simulink model "UAV_sync_known_sim_wrong_version"  (R2018b)
settings: Solver=ode23tb  StartTime=0.0  StopTime=35
values from neighbouring files (symbols this model uses):
  C_rho = 1.225    [SC42120_UAV_Preconditions.m]
  D0 = [M0 0 0 0 0 0 ... (first row only)    [SC42120_UAV_Preconditions.m]
  D1 = [eye(3)*M1 zeros(3,3) ... (first row only)    [UAV_sync_known.m]    (also in UAV_sync_unknown.m; UAV_sync_unknown_gap.m)
  D2 = [eye(3)*M2 zeros(3,3) ... (first row only)    [UAV_sync_known.m]    (also in UAV_sync_unknown.m; UAV_sync_unknown_gap.m)
  Derivative_gain_phi = 50    [SC42120_UAV_Preconditions.m]
  Derivative_gain_psi = 50    [SC42120_UAV_Preconditions.m]
  Derivative_gain_theta = 50    [SC42120_UAV_Preconditions.m]
  Derivative_gain_x = 50    [SC42120_UAV_Preconditions.m]
  Derivative_gain_y = 50    [SC42120_UAV_Preconditions.m]
  Derivative_gain_z = 50    [SC42120_UAV_Preconditions.m]
  G = 9.80665    [SC42120_UAV_Preconditions.m]
  g0 = [0;0;-M0*G;0;0;0]    [SC42120_UAV_Preconditions.m]
  I0 = [0.02 0 -0.01 ... (first row only)    [SC42120_UAV_Preconditions.m]
  I1 = [0.1 0 -0.01 ... (first row only)    [UAV_sync_known.m]    (also in UAV_sync_unknown.m; UAV_sync_unknown_gap.m)
  I2 = 2*[0.1 0 -0.01 ... (first row only)    [UAV_sync_known.m]    (also in UAV_sync_unknown.m; UAV_sync_unknown_gap.m)
  InitWind = [0;0;0]    [SC42120_UAV_Preconditions.m]
  Kp = diag(P)    [SC42120_UAV_Preconditions.m]
  Kv = diag(V)    [SC42120_UAV_Preconditions.m]
  M0 = 10    [SC42120_UAV_Preconditions.m]
  M1 = 20    [UAV_sync_known.m]    (also in UAV_sync_unknown.m; UAV_sync_unknown_gap.m)
  M2 = 30    [UAV_sync_known.m]    (also in UAV_sync_unknown.m; UAV_sync_unknown_gap.m)
  Proportional_phi = 50    [SC42120_UAV_Preconditions.m]
  Proportional_psi = 50    [SC42120_UAV_Preconditions.m]
  Proportional_theta = 50    [SC42120_UAV_Preconditions.m]
  Proportional_x = 50    [SC42120_UAV_Preconditions.m]
  Proportional_y = 50    [SC42120_UAV_Preconditions.m]
  Proportional_z = 50    [SC42120_UAV_Preconditions.m]
undefined symbols (not defined in the file or in its folder): Aero, APlane, Bxl, C, Ctr, deg, DiscIntNeverNeededParam, F, Guid, Init, Light, MIL, Path, rad, s, Trim, Utility
libraries: aerolibconvert2 x37, simulink x15, dspsigops x7, shared6dof x4, aerolibasang x4, sharedutil x4, simulink_extras x3, aerolibadyn x1, aerolibtransform2 x1, aerolibwind2 x1
(part 6 of 6)

== matlab function UAV_sync_known_sim_wrong_version/Node 0/VF Approach/AUTOPILOT/Low-level Controllers/Pitch controller/TRASH/Pitch_PID_MATLAB_Fcn ==
  data: desired_rate input; meas_pitch_rate input; out output; meas_roll_angle input; scaler input; aspeed input; time input; parteInt output; parteDer output; parteFF output; parteP output; parameters input
function [out, parteInt, parteDer, parteFF, parteP] = pitch_rate_controller...
    (desired_rate, meas_pitch_rate, meas_roll_angle, scaler, aspeed, time, ... % inputs
    parameters) % parameters
%%

gainstau = parameters(1);
gainsP = parameters(2);
gainsI = parameters(3);
gainsD = parameters(4);
gainsimax = parameters(5);
gainsFF = parameters(6);
airspeed_min = parameters(7);
eas2tas = parameters(8);
roll_limit = parameters(9);

persistent last_t;
persistent last_out;
persistent pidInfoI;

if isempty(last_t)
    last_t = 0;
end

if isempty(pidInfoI)
    pidInfoI = 0;
end

if isempty(last_out)
    last_out = 0;
end

if time==0
    last_t = 0;
    last_out=0;
    pidInfoI=0;
end

%% Start of code

tnow = time;
dt = tnow - last_t;

if (last_t == 0 || dt > 1)
    dt = 0;
end

last_t = tnow;

delta_time = dt; % * 0.001; Because the microcontroller gives [ms] - REMOVED

achieved_rate = meas_pitch_rate;
rate_error = rad2deg((desired_rate - achieved_rate) * scaler);

if gainsI > 0
    k_I = gainsI;
        if (gainsFF == 0)
    %                     /*
    %               if the user hasn't set a direct FF then assume they are
    %               not doing sophisticated tuning. Set a minimum I value of
    %               0.15 to ensure that the time constant for trimming in
    %               pitch is not too long. We have had a lot of user issues
    %               with very small I value leading to very slow pitch
    %               trimming, which causes a lot of problems for TECS. A
    %               value of 0.15 is still quite small, but a lot better
    %               than what many users are running.
    %              */
            k_I = max(k_I, 0.15);
        end
    ki_rate = k_I * gainstau;
    %     only integrate if gain and time step are positive and airspeed above min value.
    if (dt > 0 && aspeed > 0.5*airspeed_min)
        integrator_delta = rate_error * ki_rate * delta_time * scaler;
        if last_out < -45
            %              prevent the integrator from increasing if surface defln demand is above the upper limit
            integrator_delta = max(integrator_delta, 0);
        elseif last_out > 45
            %             prevent the integrator from decreasing if surface defln demand  is below the lower limit
            integrator_delta = min(integrator_delta, 0);
        end
        pidInfoI = pidInfoI + integrator_delta;
    end
else
    pidInfoI = 0;
end

intLimScaled = gainsimax * 0.01;
pidInfoI = constrain_value(pidInfoI, -intLimScaled, intLimScaled);


% get ESTIMATED to TRUE airspeed ratio (assuming 1, as in
% Airspeed_calibration.cpp)

% Calculate equivalent gains so that values for K_P and K_I can be taken across from the old PID law
% No conversion is required for K_D
kp_ff = max((gainsP - gainsI * gainstau) * gainstau  - gainsD , 0) / eas2tas;
k_ff = gainsFF / eas2tas;

% Calculate the demanded control surface deflection
% Note the scaler is applied again. We want a 1/speed scaler applied to the feed-forward
% path, but want a 1/speed^2 scaler applied to the rate error path.
% This is because acceleration scales with speed^2, but rate scales with speed.
pidInfoD = rate_error * gainsD * scaler;
pidInfoP = desired_rate * kp_ff * scaler;
pidInfoFF = desired_rate * k_ff * scaler;
last_out = pidInfoFF + pidInfoP + pidInfoD;
% pidInfodesired = desired_rate;
last_out = last_out + pidInfoI;

% when we are past the users defined roll limit for the
% aircraft our priority should be to bring the aircraft back
% within the roll limit. Using elevator for pitch control at
% large roll angles is ineffective, and can be counter
% productive as it induces earth-frame yaw which can reduce
% the ability to roll. We linearly reduce elevator input when
% beyond the configured roll limit, reducing to zero at 90
% degrees
roll_wrapped = rad2deg(abs(meas_roll_angle));

if roll_wrapped > 90
    roll_wrapped = 180-roll_wrapped;
end
% 
% if (roll_wrapped>roll_limit+5 && roll_limit<85 && abs(meas_pitch_rate) < 70)
%     roll_prop = (roll_wrapped - (roll_limit+5) / (90-roll_limit));
%     last_out = last_out * (1 - roll_prop);
% end

out = constrain_value(last_out * 100, -4500, 4500);

parteInt = pidInfoI;
parteDer = pidInfoD;
parteFF = pidInfoFF;
parteP = pidInfoP;

== matlab function UAV_sync_known_sim_wrong_version/Node 0/VF Approach/BIXLER DYNAMICS/RUBBISH BIN/Straight Line/Vg Estimator/SL_Estimator ==
  data: chi input; chi_d input; chi_q input; e input; Vg_hat input; Vg_hat_dot output size=1; param input; e output; f1 output; f2 output; Vg input
function [Vg_hat_dot, e, f1, f2]...
    = estimator (chi, chi_d, chi_q, e, Vg_hat, param, Vg)
%  feedback, der, term2, last_term,diff_chi, diff_2,
%estimator of Vg'
%% Parameters
y_int = param(1);
W = param(2);
Va = param(3);
epsi = param(4);
phiw = param(5);
chi_inf = param(6);
k = param(7);
kk=param(8);
Gamma = param(9);
sigma = param(10);

%% Law

rho = y_int^2/pi^2;   % Positive scale factor used to weight the terms so that y and chi are similar in magnitude

diff_chi = chi-chi_d; % Error of course angle

term =diff_chi/epsi;
if abs(term)<=1
    sat=term;
else
    sat=sign(term);
end

% % derivative of Vg' over x'
der = W*sin(phiw-chi)+(Va^2-W^2*(sin(phiw-chi))^2)^(-0.5)*W^2*sin(phiw-chi)*cos(phiw-chi); % partial derivative of Vg' over chi'
% 
% % Vg2_hat_dot =-i*Gamma*rho*diff_chi*chi_inf*2/pi*(k*(sin(chi2)-a*cos(chi2)))/(1+(k*(e))^2)+der*(i*chi_inf*2/pi*(k*(sin(chi2)-a*cos(chi2)))/(1+(k*(e))^2)*Vg2_hat-kk*sat);
term2 = (-1*chi_inf*2/pi*(k*sin(chi - chi_q))/(1+(k*(e))^2)*Vg_hat);
last_term = -1*kk*sat;
f2 = (sin(chi - chi_q));
f1 =  k/(1+(k*e)^2)*Gamma*rho*diff_chi*chi_inf*2/pi;

alpha = 0.4578;

% if Vg_hat - Vg > 0.5
%     sigma = (Vg_hat - Vg);
% else
%     sigma = 0;
% end
Gamma = 5;
Vg_hat_dot = Gamma/alpha*rho*diff_chi*chi_inf*2/pi*(k*(sin(chi-chi_q)))/(1+(k*(e))^2)...
    - sigma* Gamma * Vg_hat +...
     1*der*(term2/alpha +last_term);



end

== matlab function UAV_sync_known_sim_wrong_version/Node 0/VF Approach/AUTOPILOT/Low-level Controllers/Pitch controller/TRASH/Coordination_offset_MATLAB_Fcn ==
  data: bank_angle input; rate_offset output; meas_pitch_angle input; aspeed input; parameters input; inverted output
function [rate_offset, inverted] = coord_rate_offset(bank_angle, meas_pitch_angle, aspeed, parameters)

param = [  parameters(1), parameters(2), parameters(3), parameters(4) ];
[rate_offset, inverted] = get_coordination_rate(bank_angle, meas_pitch_angle, aspeed, param);

== matlab function UAV_sync_known_sim_wrong_version/Node 0/VF Approach/BIXLER DYNAMICS/RUBBISH BIN/TECS/Energy calculations/Calculate energies/TAS Rate Limiter ==
  data: TS_dem_adj output; TAS_dem input; TAS_rate_dem output; velRateMax input; velRateMin input
function [TS_dem_adj, TAS_rate_dem] = RateLimiter (TAS_dem, velRateMax, velRateMin)

persistent TAS_dem_adj
persistent TAS_dem_last

TASmin = 6;
TASmax = 35;

if isempty(TAS_dem_adj)
    TAS_dem_adj = 0;
end

if isempty(TAS_dem_last)
    TAS_dem_last = 0;
end


% Apply rate limit
if ((TAS_dem - TAS_dem_adj) > (velRateMax * 0.1))
    TAS_dem_adj = TAS_dem_adj + velRateMax * 0.1;
    TAS_rate_dem = velRateMax;
elseif ((TAS_dem - TAS_dem_adj) < (velRateMin * 0.1))
    TAS_dem_adj = TAS_dem_adj + velRateMin * 0.1;
    TAS_rate_dem = velRateMin;
else
    TAS_dem_adj = TAS_dem;
    TAS_rate_dem = (TAS_dem - TAS_dem_last) / 0.1;
end
%     Constrain speed demand again to protect against bad values on initialisation.
TAS_dem_adj = constrain_value(TAS_dem_adj, TASmin, TASmax);

TS_dem_adj = TAS_dem_adj; % Output 
TAS_dem_last = TAS_dem;

== matlab function UAV_sync_known_sim_wrong_version/Node 0/VF Approach/BIXLER DYNAMICS/RUBBISH BIN/TECS/PITCH1/Integrator ==
  data: integSEB_delta input; y output; integSEB_min input; integSEB_max input
function y = fcn(integSEB_delta, integSEB_min, integSEB_max)

persistent integSEB_state

if isempty(integSEB_state)
    integSEB_state = 0;
end

integSEB_state = constrain_value(integSEB_state + integSEB_delta, integSEB_min, integSEB_max);

y = integSEB_state;

== matlab function UAV_sync_known_sim_wrong_version/Node 0/VF Approach/BIXLER DYNAMICS/RUBBISH BIN/Straight Line/Compute crosstrack error/Xtrack error ==
  data: x input; chi_q output; y input; chi input; slope input; origin input; epy output
function [chi_q, epy]= fcn(x, y, chi, slope, origin)

chi_q = atan2(slope(2),slope(1));    % Course of the straight line [rad]
 
while chi_q - chi < -pi
    chi_q = chi_q + 2*pi;
end
while chi_q - chi > pi
    chi_q = chi_q - 2*pi;
end

epy = -sin(chi_q)*(x-origin(1)) + cos(chi_q)*(y-origin(2));

== matlab function UAV_sync_known_sim_wrong_version/Node 0/VF Approach/BIXLER DYNAMICS/RUBBISH BIN/TECS/Energy calculations/Calculate energies/Height Rate limiter ==
  data: hgt_dem input; hgt_dem output; maxClimbRate input; max_sink_rate input
function hgt_dem = RateLimiter (hgt_dem, maxClimbRate,  max_sink_rate)

persistent hgt_dem_prev

if isempty(hgt_dem_prev)
    hgt_dem_prev=0;
end

if ((hgt_dem - hgt_dem_prev) > (maxClimbRate * 0.1))
    hgt_dem = hgt_dem_prev + maxClimbRate * 0.1;
elseif ((hgt_dem - hgt_dem_prev) < (-max_sink_rate * 0.1))
    hgt_dem = hgt_dem_prev - max_sink_rate * 0.1;
end

hgt_dem_prev = hgt_dem;

== matlab function UAV_sync_known_sim_wrong_version/Node 0/VF Approach/BIXLER DYNAMICS/RUBBISH BIN/TECS/PITCH/PitchRateLimiter ==
  data: pitch_dem input; pitch_dem output; ptchRateIncr input
function pitch_dem = rateLimiter(pitch_dem, ptchRateIncr)

persistent last_pitch_dem

if isempty(last_pitch_dem)
    last_pitch_dem = 0;
end

if ((pitch_dem - last_pitch_dem) > ptchRateIncr)
    pitch_dem = last_pitch_dem + ptchRateIncr;
elseif ((pitch_dem - last_pitch_dem) < -ptchRateIncr)
    pitch_dem = last_pitch_dem - ptchRateIncr;
end
last_pitch_dem = pitch_dem;

== matlab function UAV_sync_known_sim_wrong_version/Node 0/VF Approach/BIXLER DYNAMICS/RUBBISH BIN/TECS/PITCH/MATLAB Function ==
  data: temp input; integSEB_delta output; gainInv input; PITCHminf input; PITCHmaxf input; integSEB_delta input; integSEB_min output; integSEB_max output
function [integSEB_delta, integSEB_min, integSEB_max] = integSEB(temp, gainInv, PITCHminf, PITCHmaxf, integSEB_delta )


integSEB_min = (gainInv * (PITCHminf - 0.0783)) - temp;
integSEB_max = (gainInv * (PITCHmaxf + 0.0783)) - temp;
integSEB_range = integSEB_max - integSEB_min;

    
% don't allow the integrator to rise by more than 20% of its full
% range in one step. This prevents single value glitches from
% causing massive integrator changes. See Issue#4066

integSEB_delta = constrain_value(integSEB_delta, -integSEB_range*0.1, integSEB_range*0.1);

== matlab function UAV_sync_known_sim_wrong_version/Node 0/VF Approach/BIXLER DYNAMICS/RUBBISH BIN/Orbit/Chi_d/Vector Field (loiter) ==
  data: gamma input; j input; d input; radius input; k input; chi_d output; d_tilde output
function [chi_d, d_tilde]  = VF_method( gamma, j, d, radius, k )

d_tilde = d-radius;
chi_d = gamma + j*(pi/2 + atan(k*d_tilde));


% 
% positiveInput = (chi_d > 0);
% chi_d = mod(chi_d, 2*pi);
% chi_d((chi_d == 0) & positiveInput) = 2*pi;

% q = (chi_d < -pi) | (pi < chi_d);
% arg = chi_d(q) + pi;
% positiveInput = (arg > 0);
% arg = mod(arg, 2*pi);
% arg((arg == 0) & positiveInput) = 2*pi;
% chi_d(q) = arg - pi;
end

== matlab function UAV_sync_known_sim_wrong_version/Node 0/VF Approach/BIXLER DYNAMICS/RUBBISH BIN/Straight Line/SL.controller/SL.Controller ==
  data: chi input; chi_d input; e input; Vg_hat input; chi_q input; chi_c output; param input
function chi_c = CommandCourse(chi,chi_d,e,Vg_hat, chi_q, param)
%generate command course angle chi_c
%% Params
epsi = param(1);
chi_inf = param(2);
k = param(3);
kk = param(4);
alpha = param(5);

%% Controller

term =(chi-chi_d)/epsi;
if abs(term)<=1
    chi_tilde_norm = term;
else
    chi_tilde_norm = sign(term);
end

% chi_c=chi2 + ...
%     i*chi_inf*2/pi/alpha*(k*(sin(chi2)-a*cos(chi2)))/(1+(k*(e))^2)*(Vg2_hat)-kk/alpha*sat;

% term1 = chi;
% term2 = -1*chi_inf*2/pi/alpha*k*(sin(chi-chi_q))/(1+(k*(e))^2)*Vg_hat;
% term3 = -kk/alpha*chi_tilde_norm;

% chi_c= term1 + term2 + term3;

chi_c=chi - chi_inf*2/pi/alpha*(k* sin(chi - chi_q))/(1+(k*(e))^2)*(Vg_hat)-kk/alpha*chi_tilde_norm;
 

end

== matlab function UAV_sync_known_sim_wrong_version/Node 0/VF Approach/BIXLER DYNAMICS/RUBBISH BIN/Straight Line/Chi_d/Vector Field (straight line) ==
  data: e_y input; chi_d output; chi_q input; chi_inf input; k_line input
function chi_d   = VF_method(e_y, chi_q, chi_inf, k_line )

term2 = -1 * chi_inf * 2/pi * atan(k_line * e_y);
chi_d = chi_q + term2; % Vector field law

end

== matlab function UAV_sync_known_sim_wrong_version/Node 0/VF Approach/BIXLER DYNAMICS/RUBBISH BIN/Straight Line/SL.controller/Beard version ==
  data: chi input; chi_d input; e input size=1; Vg input; chi_c output; param input; chi_q input
function chi_c  = CommandCourse(chi,chi_d,e,Vg,param,chi_q)
%generate command course angle chi_c

%% Parameters
epsi = param(1);
chi_inf = param(2);
k = param(3);
kk = param(4);
alpha = param(5);

%%
term =(chi-chi_d)/epsi;
if abs(term)<=1
    chi_tilde_norm=term;
else
    chi_tilde_norm=sign(term);
end

term1 = chi;
term2 = -1*chi_inf*2/pi/alpha*k*(sin(chi-chi_q))/(1+(k*(e))^2)*Vg;
term3 = -kk/alpha*chi_tilde_norm;

chi_c= term1 + term2 + term3;
% 
% chi_c= chi -1 *chi_inf*2/pi/alpha*k*(sin(chi)*cos(chi_q)-cos(chi)*sin(chi_q))/(1+(k*(e))^2)*Vg...
%      -kk/alpha*sat;
% chi_c=chi + ...
%     i*chi_inf*2/pi/alpha* (k/(1+(k*e)^2))*Vg*sin(chi)-kk/alpha*sat;
% 
end

== matlab function UAV_sync_known_sim_wrong_version/Node 0/VF Approach/BIXLER DYNAMICS/RUBBISH BIN/TECS/THROTTLE/Throttle Integrator ==
  data: throttle_dem input; throttle_dem output; THRminf input; THRmaxf input; throttle_slewrate input; K_STE2Thr input; STE_error input; integGain input; DT input
function throttle_dem = ThrottleIntegrator(throttle_dem, THRminf, THRmaxf, throttle_slewrate,...
                                K_STE2Thr,STE_error,integGain,...
                                DT)

persistent last_throttle_dem
persistent integTHR_state

if isempty(last_throttle_dem)
    last_throttle_dem = 0;
end

if isempty(integTHR_state)
    integTHR_state = 0;
end

THRminf_clipped_to_zero = constrain_value(THRminf, 0, THRmaxf);

%Rate limit PD + FF throttle
%Calculate the throttle increment from the specified slew time
if (throttle_slewrate ~= 0)
    thrRateIncr = DT * (THRmaxf - THRminf_clipped_to_zero) * throttle_slewrate * 0.01;
    throttle_dem = constrain_value(throttle_dem,...
        last_throttle_dem - thrRateIncr,...
        last_throttle_dem + thrRateIncr);
    last_throttle_dem = throttle_dem;
end

%Calculate integrator state upper and lower limits
%Set to a value that will allow 0.1 (10%) throttle saturation to allow for noise on the demand
%Additionally constrain the integrator state amplitude so that the integrator comes off limits faster.
maxAmp = 0.5 * (THRmaxf - THRminf_clipped_to_zero);
integ_max = constrain_value((THRmaxf - throttle_dem + 0.1),-maxAmp,maxAmp);
integ_min = constrain_value((THRminf - throttle_dem - 0.1),-maxAmp,maxAmp);

%Calculate integrator state, constraining state
%Set integrator to a max throttle value during climbout
integTHR_state = integTHR_state + (STE_error * integGain) * DT * K_STE2Thr;

integTHR_state = constrain_value(integTHR_state, integ_min, integ_max);

%Sum the components.
throttle_dem = throttle_dem + integTHR_state;

% Constrain throttle demand
throttle_dem = constrain_value(throttle_dem, THRminf, THRmaxf);

== matlab function UAV_sync_known_sim_wrong_version/Node 0/VF Approach/BIXLER DYNAMICS/RUBBISH BIN/Orbit/Vg Estimator/Estimator  ==
  data: chi input; d input; Vg2_hat_dot output size=1; Vg_hat input; gamma input; chi_d input; param input; beta output; der output; term1 output; term2 output; err_1 output; err_2 output; chi_tilde output; Vg input
function [Vg2_hat_dot, beta, der, term1, term2, err_1, err_2, chi_tilde] = estimator(chi,d,Vg_hat,gamma,chi_d, param, Vg)

%% Parameters
W = param(1);
phiw = param(2);
Va  = param(3);
k  = param(4);
kk = param(5);
epsi = param(6);
d_int = param(7);
R  = param(8);
j = param(9);
Gamma = param(10);
sigma = param(11);

%% Estimator of Vg'

err_1 = (phiw - chi);
err_2 = chi - gamma;
chi_tilde = chi - chi_d;

term = chi_tilde / epsi;
rho = (d_int / pi)^2;

if abs(term) <= 1
    chi_tilde_eps = term;
else
    chi_tilde_eps = sign(term);
end

if Vg_hat - Vg > 0.5
    sigma = (Vg_hat - Vg);
else
    sigma = 0;
end


% Partial derivative of Vg' over chi'
beta = k/(1 + (k * (d - R))^2);
der = W * sin(err_1) + (Va^2 - W^2 * (sin(err_1))^2)^(-0.5) * W^2 * sin(err_1) * cos(err_1); 

term1 = -Gamma * rho * (chi_tilde) * (sin(err_2) / d + j * beta * cos(err_2));
term2 = der*(Vg_hat*sin(err_2)/d + j*beta*Vg_hat*cos(err_2) - kk*chi_tilde_eps);
Vg2_hat_dot =  term1 + 1*term2 - sigma*Gamma*Vg_hat;
end

== matlab function UAV_sync_known_sim_wrong_version/Node 0/VF Approach/BIXLER DYNAMICS/RUBBISH BIN/Orbit/Compute gamma/L.PolarCoord ==
  data: x input; y input; gamma output; c input; d output; chi input
function [gamma, d] = pol_coord(x,y,c,chi)
p = [x,y];
d = sqrt((p(1)-c(1))^2+(p(2)-c(2))^2);
gamma = atan2(p(2)-c(2),p(1)-c(1));

% while gamma - chi < -pi
%     gamma = gamma + 2*pi;
% end
% 
% while gamma - chi > pi
%     gamma = gamma - 2*pi;
% end

end

== matlab function UAV_sync_known_sim_wrong_version/Node 0/VF Approach/BIXLER DYNAMICS/RUBBISH BIN/TECS/PITCH/Integrator ==
  data: integSEB_delta input; y output; integSEB_min input; integSEB_max input
function y = fcn(integSEB_delta, integSEB_min, integSEB_max)

persistent integSEB_state

if isempty(integSEB_state)
    integSEB_state = 0;
end

integSEB_state = constrain_value(integSEB_state + integSEB_delta, integSEB_min, integSEB_max);

y = integSEB_state;

== matlab function UAV_sync_known_sim_wrong_version/Node 0/VF Approach/BIXLER DYNAMICS/RUBBISH BIN/Orbit/Loiter Controller/Loiter Controller ==
  data: chi input; y output; chi_d input; d input; Vg input; gamma input; err output; beta output; term2 output; param input; term3 output
function [y, err, beta, term2, term3] = OrbitController(chi, chi_d, d, Vg, gamma, param)

%%
k = param(1);
kk = param(2);
epsi = param(3);
r = param(4);
j = param(5);
alpha = param(6);

%%
chi_tilde = chi-chi_d;
lt = chi_tilde/epsi;

if abs(lt) <=1
    term = lt;
else
    term = sign(lt);
end

d_tilde = d-r;
beta = k/(1+(k*d_tilde)^2);

err = (chi-gamma);

term2 = Vg /(alpha*d)*sin(err) + j*beta/alpha*Vg*cos(err);

term3 = -kk/alpha*term;

y = chi + term2 + term3;

== matlab function UAV_sync_known_sim_wrong_version/Node 0/VF Approach/BIXLER DYNAMICS/RUBBISH BIN/Vector Field ==
  data: y output; y input
function y = VF_method(y)

chi_inf = 70;                   %degrees
chi_inf = deg2rad(chi_inf);
k = 0.08;                       %tuning paremeter

psi_demanded = -chi_inf * 2 / pi * atan2(k*y, 1);

y = rad2deg(psi_demanded);

== matlab function UAV_sync_known_sim_wrong_version/Node 0/VF Approach/PATH FOLLOWING/Orbit Path Following (Enabled Subsystem)/Compute gamma and distance to center/MATLAB Function ==
  data: gamma input; gamma output; chi input
function gamma = fcn(gamma, chi)

while gamma - chi < -pi
    gamma = gamma + 2*pi;
end
while gamma - chi > pi
    gamma = gamma - 2*pi;
end

== matlab function UAV_sync_known_sim_wrong_version/Node 0/VF Approach/BIXLER DYNAMICS/RUBBISH BIN/Straight Line/..Ground velocity ==
  data: chi input; Vg output; w input; phiw input; Va input
function Vg = GroundVelocity(chi,w,phiw,Va)
%generate the ground velocity based on course angle
Vg=w*cos(chi-phiw)+sqrt(Va^2-w^2*(sin(chi-phiw))^2);
end

== matlab function UAV_sync_known_sim_wrong_version/Node 0/VF Approach/BIXLER DYNAMICS/Vehicle Airframe/to Omega_e/MATLAB Function ==
  data: attitude input; omega_e output; omega_b input
function omega_e   = fromBODYtoNEDangvel( attitude, omega_b )

phi = attitude(1);
theta = attitude(2);

E_inv = [1 sin(phi)*tan(theta), cos(phi)*tan(theta); 
     0 cos(phi) -sin(phi);
     0 -sin(phi)/cos(theta) cos(phi)/cos(theta)];

omega_e = E_inv * omega_b;     

end

== matlab function UAV_sync_known_sim_wrong_version/Node 0/VF Approach/BIXLER DYNAMICS/RUBBISH BIN/TECS/PITCH1/MATLAB Function ==
  data: temp input; integSEB_delta output; gainInv input; PITCHminf input; PITCHmaxf input; integSEB_delta input; integSEB_min output; integSEB_max output
function [integSEB_delta, integSEB_min, integSEB_max] = integSEB(temp, gainInv, PITCHminf, PITCHmaxf, integSEB_delta )


integSEB_min = (gainInv * (PITCHminf - 0.0783)) - temp;
integSEB_max = (gainInv * (PITCHmaxf + 0.0783)) - temp;
integSEB_range = integSEB_max - integSEB_min;

    
% don't allow the integrator to rise by more than 20% of its full
% range in one step. This prevents single value glitches from
% causing massive integrator changes. See Issue#4066

integSEB_delta = constrain_value(integSEB_delta, -integSEB_range*0.1, integSEB_range*0.1);

== matlab function UAV_sync_known_sim_wrong_version/Node 0/VF Approach/BIXLER DYNAMICS/RUBBISH BIN/TECS/PITCH1/PitchRateLimiter ==
  data: pitch_dem input; pitch_dem output; ptchRateIncr input
function pitch_dem = rateLimiter(pitch_dem, ptchRateIncr)

persistent last_pitch_dem

if isempty(last_pitch_dem)
    last_pitch_dem = 0;
end

if ((pitch_dem - last_pitch_dem) > ptchRateIncr)
    pitch_dem = last_pitch_dem + ptchRateIncr;
elseif ((pitch_dem - last_pitch_dem) < -ptchRateIncr)
    pitch_dem = last_pitch_dem - ptchRateIncr;
end
last_pitch_dem = pitch_dem;

== matlab function UAV_sync_known_sim_wrong_version/Node 0/VF Approach/BIXLER DYNAMICS/RUBBISH BIN/TECS/THROTTLE1/MATLAB Function ==
  data: throttle_dem input; throttle_dem output; THRminf input; THRmaxf input; throttle_slewrate input; K_STE2Thr input; STE_error input; integGain input; DT input
function throttle_dem = ThrottleIntegrator(throttle_dem, THRminf, THRmaxf, throttle_slewrate,...
                                K_STE2Thr,STE_error,integGain,...
                                DT)

persistent last_throttle_dem
persistent integTHR_state

if isempty(last_throttle_dem)
    last_throttle_dem = 0;
end

if isempty(integTHR_state)
    integTHR_state = 0;
end

THRminf_clipped_to_zero = constrain_value(THRminf, 0, THRmaxf);

%Rate limit PD + FF throttle
%Calculate the throttle increment from the specified slew time
if (throttle_slewrate ~= 0)
    thrRateIncr = DT * (THRmaxf - THRminf_clipped_to_zero) * throttle_slewrate * 0.01;
    throttle_dem = constrain_value(throttle_dem,...
        last_throttle_dem - thrRateIncr,...
        last_throttle_dem + thrRateIncr);
    last_throttle_dem = throttle_dem;
end

%Calculate integrator state upper and lower limits
%Set to a value that will allow 0.1 (10%) throttle saturation to allow for noise on the demand
%Additionally constrain the integrator state amplitude so that the integrator comes off limits faster.
maxAmp = 0.5 * (THRmaxf - THRminf_clipped_to_zero);
integ_max = constrain_value((THRmaxf - throttle_dem + 0.1),-maxAmp,maxAmp);
integ_min = constrain_value((THRminf - throttle_dem - 0.1),-maxAmp,maxAmp);

%Calculate integrator state, constraining state
%Set integrator to a max throttle value during climbout
integTHR_state = integTHR_state + (STE_error * integGain) * DT * K_STE2Thr;

integTHR_state = constrain_value(integTHR_state, integ_min, integ_max);

%Sum the components.
throttle_dem = throttle_dem + integTHR_state;

% Constrain throttle demand
throttle_dem = constrain_value(throttle_dem, THRminf, THRmaxf);

== matlab function UAV_sync_known_sim_wrong_version/Node 0/VF Approach/BIXLER DYNAMICS/RUBBISH BIN/TECS/PITCH/Integrator1 ==
  data: integSEB_delta input; y output; integSEB_min input; integSEB_max input
function y = fcn(integSEB_delta, integSEB_min, integSEB_max)

persistent integSEB_state

if isempty(integSEB_state)
    integSEB_state = 0;
end

integSEB_state = constrain_value(integSEB_state + integSEB_delta, integSEB_min, integSEB_max);

y = integSEB_state;

== matlab function UAV_sync_known_sim_wrong_version/Node 0/VF Approach/PATH FOLLOWING/Straight-line Path Following (Enabled Subsystem)/Chi_d/Vector Field (straight line) ==
  data: e_y input; chi_d output; chi_q input; chi_inf input; k_line input
function chi_d   = VF_method(e_y, chi_q, chi_inf, k_line )

term2 = -1 * chi_inf * 2/pi * atan(k_line * e_y);
chi_d = chi_q + term2; % Vector field law

end

== matlab function UAV_sync_known_sim_wrong_version/Node 0/VF Approach/PATH FOLLOWING/Straight-line Path Following (Enabled Subsystem)/Compute crosstrack error/chi_q_correction ==
  data: chi_q input; chi_q output; chi input
function chi_q = fcn(chi_q, chi)

while chi_q - chi < -pi
    chi_q = chi_q + 2*pi;
end
while chi_q - chi > pi
    chi_q = chi_q - 2*pi;
end

== matlab function UAV_sync_known_sim_wrong_version/Node 0/VF Approach/PATH FOLLOWING/Straight-line Path Following (Enabled Subsystem)/SL.controller/SL.Controller ==
  data: chi input; chi_d input; e input size=1; Vg input; chi_c output; param input; chi_q input
function chi_c  = CommandCourse(chi,chi_d,e,Vg,param,chi_q)
%generate command course angle chi_c

%% Parameters
epsi = param(1);
chi_inf = param(2);
k = param(3);
kk = param(4);
alpha = param(5);

%%
term =(chi-chi_d)/epsi;
if abs(term)<=1
    chi_tilde_norm=term;
else
    chi_tilde_norm=sign(term);
end

term1 = chi;
term2 = -1*chi_inf*2/pi/alpha*k*(sin(chi-chi_q))/(1+(k*(e))^2)*Vg;
term3 = -kk/alpha*chi_tilde_norm;

chi_c= term1 + term2 + term3;
 
end

== matlab function UAV_sync_known_sim_wrong_version/Node 0/VF Approach/PATH FOLLOWING/Straight-line Path Following (Enabled Subsystem)/Vg Estimator/SL_Estimator ==
  data: chi input; chi_d input; chi_q input; e input; param input; Vg input; Vg_hat input; Vg_hat_dot output size=1
function Vg_hat_dot ...
    = estimator (chi, chi_d, chi_q, e, param, Vg, Vg_hat)
%  feedback, der, term2, last_term,diff_chi, diff_2,
%estimator of Vg'
%% Parameters
y_int = param(1);
W = param(2);
Va = param(3);
epsi = param(4);
phiw = param(5);
chi_inf = param(6);
k = param(7);
kk=param(8);
Gamma = param(9);
sigma = param(10);
alpha = param(11);

%% Law

rho = y_int^2/pi^2;   % Positive scale factor used to weight the terms so that y and chi are similar in magnitude

diff_chi = chi-chi_d; % Error of course angle

term =diff_chi/epsi;
if abs(term)<=1
    sat=term;
else
    sat=sign(term);
end

% % derivative of Vg' over x'
der = W*sin(phiw-chi)+(Va^2-W^2*(sin(phiw-chi))^2)^(-0.5)*W^2*sin(phiw-chi)*cos(phiw-chi); % partial derivative of Vg' over chi'

term2 = (-1*chi_inf*2/pi*(k*sin(chi - chi_q))/(1+(k*(e))^2)*Vg_hat);
last_term = -1*kk*sat;

% if Vg_hat - Vg > 1
%     sigma = (Vg_hat - Vg);
% else
%     sigma = 0;
% end

Vg_hat_dot = Gamma/alpha*rho*diff_chi*chi_inf*2/pi*(k*(sin(chi-chi_q)))/(1+(k*(e))^2)...
    - sigma* Gamma * Vg_hat +...
     1*der*(term2/alpha +last_term);



end

== matlab function UAV_sync_known_sim_wrong_version/Node 0/VF Approach/PATH FOLLOWING/Orbit Path Following (Enabled Subsystem)/Compute gamma and distance to center/L.PolarCoord ==
  data: x input; y input; gamma output; c input; d output; chi input
function [gamma, d] = pol_coord(x,y,c,chi)
p = [x,y];
d = sqrt((p(1)-c(1))^2+(p(2)-c(2))^2);
gamma = atan2(p(2)-c(2),p(1)-c(1));

% while gamma - chi < -pi
%     gamma = gamma + 2*pi;
% end
% 
% while gamma - chi > pi
%     gamma = gamma - 2*pi;
% end

end

== matlab function UAV_sync_known_sim_wrong_version/Node 0/VF Approach/PATH MANAGER/Enabled Subsystem/Path Manager ==
  settings: updateMethod=DISCRETE
  data: w input; flag output; x input; y input; origin output; slope output; c output; lambda output; stop_sim output; R input
function [ flag, origin, slope, c, lambda, stop_sim] = fcn( w, x, y, R )
%%
% Index of the current waypoint
persistent i
if isempty(i)
    i = 2;
end
% State = 1 if straight line, state = 2 if orbit
persistent state
if isempty(state)
    state = 1;
end

% Init
n = size(w,1);      % Number of waypoints
flag = 1;           % Switch from SL to orbit
origin = [0 0];
slope = [1 0];
c = [0 0];
lambda = 0;
stop_sim = 0;
z=[0 0];

%%
p = [x y];
q_i_min_1 = (w(i,:)-w(i-1,:)) / norm(w(i,:)-w(i-1,:),2);
q_i = (w(i+1,:)-w(i,:)) / norm(w(i+1,:)-w(i,:),2);
rho = acos(-q_i_min_1*q_i');

if state == 1
    flag = 1;
    origin = w(i-1,:);
    slope = q_i_min_1;
    z = w(i,:) - (R/(tan(rho/2)))*q_i_min_1;
    if (p-z) * q_i_min_1' >= 0
        state = 2;
        %         i=i+1;
    end
    
elseif state == 2
    flag = 0;
    c = w(i,:)-(R/(sin(rho/2)))*(q_i_min_1 - q_i)/(norm(q_i_min_1- q_i));
    %     rho = R;
    lambda = sign(q_i_min_1(1) * q_i(2) - q_i_min_1(2)*q_i(1));
    z = w(i,:) + (R/(tan(rho/2)))*q_i;
    if (p-z) * q_i' >= 0
        i = i + 1;
        state = 1;
    end
end
if i == n-1
    stop_sim = 1;
end

end

== matlab function UAV_sync_known_sim_wrong_version/Node 0/VF Approach/PATH FOLLOWING/Orbit Path Following (Enabled Subsystem)/Loiter Controller/Loiter Controller ==
  data: chi input; y output; chi_d input; d input; Vg input; gamma input; param input
function y  = OrbitController(chi, chi_d, d, Vg, gamma, param)

%%
k = param(1);
kk = param(2);
epsi = param(3);
r = param(4);
j = param(5);
alpha = param(6);

%%
chi_tilde = chi-chi_d;
lt = chi_tilde/epsi;

if abs(lt) <=1
    term = lt;
else
    term = sign(lt);
end

d_tilde = d-r;
beta = k/(1+(k*d_tilde)^2);

err = (chi-gamma);

term2 = Vg /(alpha*d)*sin(err) + j*beta/alpha*Vg*cos(err);

term3 = -kk/alpha*term;

y = chi + term2 + term3;

== matlab function UAV_sync_known_sim_wrong_version/Node 0/VF Approach/PATH FOLLOWING/Orbit Path Following (Enabled Subsystem)/Vg Estimator/Estimator  ==
  data: chi input; d input; gamma input; chi_d input; param input; Vg input; Vg2_hat_dot output size=1; Vg_hat input
function Vg2_hat_dot  = estimator(chi,d,gamma,chi_d, param, Vg, Vg_hat)

%% Parameters
W = param(1);
phiw = param(2);
Va  = param(3);
k  = param(4);
kk = param(5);
epsi = param(6);
d_int = param(7);
R  = param(8);
j = param(9);
Gamma = param(10);
sigma = param(11);

%% Estimator of Vg'

err_1 = (phiw - chi);
err_2 = chi - gamma;
chi_tilde = chi - chi_d;

term = chi_tilde / epsi;
rho = (d_int / pi)^2;

if abs(term) <= 1
    chi_tilde_eps = term;
else
    chi_tilde_eps = sign(term);
end

if Vg_hat - Vg > 0.5 ||  Vg_hat - Vg < -0.5
    sigma = 3*(Vg_hat - Vg);
else
    sigma = 0;
end


% Partial derivative of Vg' over chi'
beta = k/(1 + (k * (d - R))^2);
der = W * sin(err_1) + (Va^2 - W^2 * (sin(err_1))^2)^(-0.5) * W^2 * sin(err_1) * cos(err_1); 

term1 = -Gamma * rho * (chi_tilde) * (sin(err_2) / d + j * beta * cos(err_2));
term2 = der*(Vg_hat*sin(err_2)/d + j*beta*Vg_hat*cos(err_2) - kk*chi_tilde_eps);
Vg2_hat_dot =  term1 + 1*term2 - sigma*Gamma*Vg_hat;
end
